simulink model "MotorControl"  (R2018b)
settings: Solver=FixedStepAuto  StartTime=0.0  StopTime=0.8  FixedStep=0.001  RelTol=1e-3  EnableMultiTasking=on
PostLoadFcn:
  | PMSM_Params
values from neighbouring files (symbols this model uses):
  Params =     [Parameters.mat]
libraries: TIMERS_Lib x3, ADC_Lib x2, USART_Lib x2, GPIO_Lib x1, STM32_Config_Lib x1
settings Model: DataTypeOverride=Double  MinMaxOverflowLogging=ForceOff  Creator=Alex  LastModifiedBy=fenard1
settings DataIOCC: LimitDataPoints=on  SaveFormat=Array
settings OptimizationCC: DefaultParameterBehavior=Inlined  DefaultUnderspecifiedDataType=single  PassReuseOutputArgsAs=Individual arguments  ExpressionDepthLimit=2147483647  LifeSpan=1
settings DebuggingCC: UnderspecifiedInitializationDetection=Classic  MergeDetectMultiDrivingBlocksExec=none  SolverPrmCheckMsg=warning  MultiTaskDSMMsg=none  UniqueDataStoreMsg=error  AllowSymbolicDim=off  StateNameClashWarn=warning  StrictBusMsg=ErrorOnBusTreatedAsVector  SFUnexpectedBacktrackingDiag=warning  SFNoUnconditionalDefaultTransitionDiag=warning  SFUndirectedBroadcastEventsDiag=error  SFExecutionAtInitializationDiag=none
settings HardwareCC: ProdBitPerPointer=32  ProdBitPerSizeT=32  ProdBitPerPtrDiffT=32  ProdLargestAtomicInteger=Integer  ProdWordSize=32  ProdHWDeviceType=STMicroelectronics->STM32 32-bit Cortex-M  TargetLargestAtomicInteger=Integer  TargetLargestAtomicFloat=Float  TargetIntDivRoundTo=Zero  TargetEndianess=LittleEndian  TargetHWDeviceType=STMicroelectronics->STM32F4xx 32-bit Cortex-M4
settings ModelReferenceCC: PropagateSignalLabelsOutOfModel=off
settings SFSimCC: SimUseLocalCustomCode=off  CompileTimeRecursionLimit=0  EnableRuntimeRecursion=off  MATLABDynamicMemAlloc=off
settings RTWCC: SystemTargetFile=stm32.tlc  TemplateMakefile=stm32.tmf  Description=stm32 (Embedded Target)  GenerateReport=on  RTWUseLocalCustomCode=off  IncludeHyperlinkInReport=on  GenerateCodeReplacementReport=on
settings CodeAppCC: IgnoreCustomStorageClasses=off  CustomSymbolStrType=$N$R$M  SimulinkBlockComments=off  InternalIdentifier=Classic
settings STFCustomTargetCC: TargetLangStandard=C99 (ISO)  CodeReplacementLibrary=ARM CMSIS SIN COS  ParMdlRefBuildCompliant=on  IncludeMdlTerminateFcn=off  CombineOutputUpdateFcns=on  ERTCustomFileBanners=on  SupportComplex=off  SupportContinuousTime=off  SupportNonInlinedSFcns=off  RemoveResetFunc=on  ParenthesesLevel=Maximum  CastingMode=Standards  MATLABClassNameForMDSCustomization=Simulink.SoftwareTarget.ERTCustomization  SystemTargetFile=stm32.tlc
settings ERTTargetCC: TargetLangStandard=C99 (ISO)  CodeReplacementLibrary=ARM CMSIS SIN COS  MultiwordLength=2048  CompOptLevelCompliant=off  ConcurrentExecutionCompliant=off  IncludeMdlTerminateFcn=off  SupportComplex=off  ParenthesesLevel=Maximum  CastingMode=Standards  ModelStepFunctionPrototypeControlCompliant=off  CPPClassGenCompliant=off  UseToolchainInfoCompliant=off  InlinedParameterPlacement=NonHierarchical  ERTSrcFileBannerTemplate=sourceFileTemplate.cgt  ERTHdrFileBannerTemplate=sourceFileTemplate.cgt  ERTDataSrcFileTemplate=sourceFileTemplate.cgt  ERTDataHdrFileTemplate=sourceFileTemplate.cgt  ERTCustomFileTemplate=customRoutineProcess.tlc  ConvertIfToSwitch=off  SuppressUnreachableDefaultCases=off  EnableSignedLeftShifts=off  EnableSignedRightShifts=off
settings ConfigComp: CovMetricSettings=dw  CovHtmlReporting=on  CovSaveCumulativeToWorkspaceVar=on  CovSaveSingleToWorkspaceVar=on  CovExternalEMLEnable=off  CovSFcnEnable=off
settings SimscapeCC: SimscapeNormalizeSystem=off

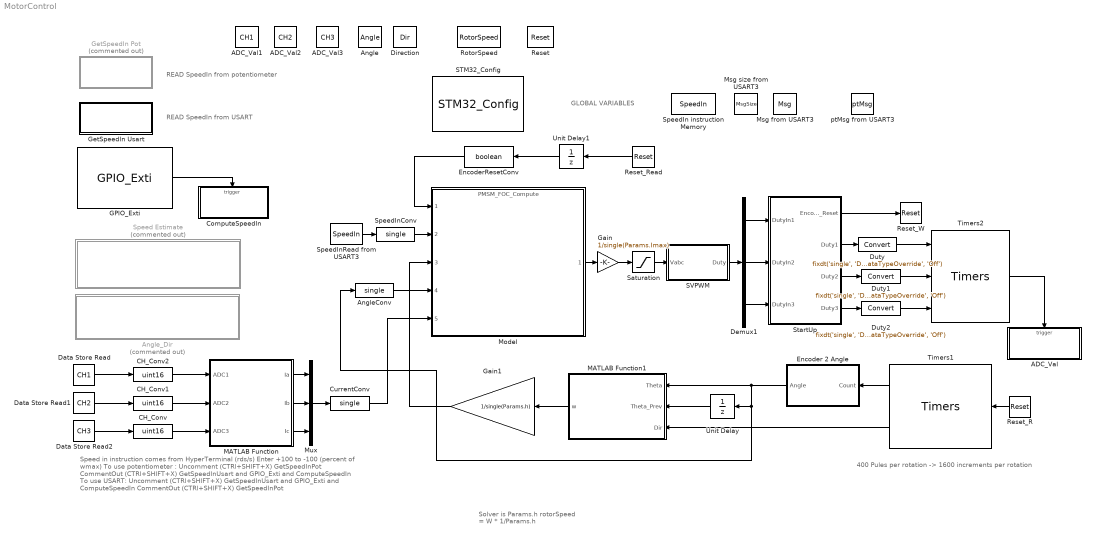
== system MotorControl ==
  note: Speed in instruction comes from HyperTerminal (rds/s)
      | Enter +100 to -100 (percent of wmax)
      | To use potentiometer :
      | Uncomment (CTRl+SHIFT+X) GetSpeedInPot
      | CommentOut (CTRl+SHIFT+X) GetSpeedInUsart and GPIO_Exti
      | and ComputeSpeedIn
      | To use USART:
      | Uncomment (CTRl+SHIFT+X) GetSpeedInUsart and GPIO_Exti
      | and ComputeSpeedIn
      | CommentOut (CTRl+SHIFT+X) GetSpeedInPot
  note: GLOBAL VARIABLES
  note: READ SpeedIn from potentiometer
  note: READ SpeedIn from USART
  note: 400 Pules per rotation -> 1600 increments per rotation
  note: Solver is Params.h
      | rotorSpeed = W * 1/Params.h
  ADC_Val : Subsystem  TreatAsAtomicUnit=on
  ADC_Val1 : DataStoreMemory  DataStoreName=CH1  ReadBeforeWriteMsg=warning  WriteAfterWriteMsg=warning  WriteAfterReadMsg=warning  ShowAdditionalParam=off  OutMin=0  OutMax=4095  OutDataTypeStr=fixdt('uint16', 'DataTypeOverride', 'Off')
  ADC_Val2 : DataStoreMemory  DataStoreName=CH2  ReadBeforeWriteMsg=warning  WriteAfterWriteMsg=warning  WriteAfterReadMsg=warning  ShowAdditionalParam=off  OutMin=0  OutMax=4095  OutDataTypeStr=fixdt('uint16', 'DataTypeOverride', 'Off')
  ADC_Val3 : DataStoreMemory  DataStoreName=CH3  ReadBeforeWriteMsg=warning  WriteAfterWriteMsg=warning  WriteAfterReadMsg=warning  ShowAdditionalParam=off  OutMin=0  OutMax=4095  OutDataTypeStr=fixdt('uint16', 'DataTypeOverride', 'Off')
  Angle : DataStoreMemory  DataStoreName=Angle  ReadBeforeWriteMsg=warning  WriteAfterWriteMsg=warning  WriteAfterReadMsg=warning  ShowAdditionalParam=off  OutDataTypeStr=fixdt('single', 'DataTypeOverride', 'Off')
  AngleConv : DataTypeConversion  OutDataTypeStr=single
  Angle_Dir : Subsystem  Commented=on  TreatAsAtomicUnit=on  SystemSampleTime=0.001
  CH_Conv : DataTypeConversion  OutDataTypeStr=uint16
  CH_Conv1 : DataTypeConversion  OutDataTypeStr=uint16
  CH_Conv2 : DataTypeConversion  OutDataTypeStr=uint16
  ComputeSpeedIn : Subsystem  TreatAsAtomicUnit=on
  CurrentConv : DataTypeConversion  OutDataTypeStr=single
  Data Store Read : DataStoreRead  DataStoreName=CH1
  Data Store Read1 : DataStoreRead  DataStoreName=CH2
  Data Store Read2 : DataStoreRead  DataStoreName=CH3
  Demux1 : Demux  Outputs=3
  Direction : DataStoreMemory  DataStoreName=Dir  ReadBeforeWriteMsg=warning  WriteAfterWriteMsg=warning  WriteAfterReadMsg=warning  ShowAdditionalParam=off  OutDataTypeStr=fixdt('uint8', 'DataTypeOverride', 'Off')
  Duty : DataTypeConversion  OutDataTypeStr=fixdt('single', 'DataTypeOverride', 'Off')
  Duty1 : DataTypeConversion  OutDataTypeStr=fixdt('single', 'DataTypeOverride', 'Off')
  Duty2 : DataTypeConversion  OutDataTypeStr=fixdt('single', 'DataTypeOverride', 'Off')
  Encoder 2 Angle : MATLAB Function  TreatAsAtomicUnit=on
      settings: MinAlgLoopOccurrences=on
  EncoderResetConv : DataTypeConversion  OutDataTypeStr=boolean
  GPIO_Exti : GPIO_Lib/GPIO_Exti  Port_name=GPIOB  Pin_0=off  Pin_1=off  Pin_2=off  Pin_3=off  Pin_4=off  Pin_5=off  Pin_6=off  Pin_7=off  Pin_8=off  Pin_9=off  Pin_10=off  Pin_11=off  Pin_12=off  Pin_13=off  Pin_14=off  Pin_15=on  PinList=GPIOB15GPIOC13
      settings: SourceProductName=Target Support Package - STM32 Adapter
  Gain : Gain  Gain=1/single(Params.Imax)
  Gain1 : Gain  Gain=1/single(Params.h)  OutDataTypeStr=double
  GetSpeedIn Pot : Subsystem  Commented=on  TreatAsAtomicUnit=on  SystemSampleTime=0.1
  GetSpeedIn Usart : Subsystem  TreatAsAtomicUnit=on  SystemSampleTime=0.1
  MATLAB Function : MATLAB Function  TreatAsAtomicUnit=on
  MATLAB Function1 : MATLAB Function  TreatAsAtomicUnit=on
  Model : ModelReference  ModelNameDialog=PMSM_FOC_Compute.slx  SimulationMode=Normal  ModelReferenceVersion=1.373
  Msg from USART3 : DataStoreMemory  DataStoreName=Msg  ReadBeforeWriteMsg=warning  WriteAfterWriteMsg=warning  WriteAfterReadMsg=warning  InitialValue=[0,0,0,0,0,0,0,0]  ShowAdditionalParam=off  OutDataTypeStr=fixdt('uint8', 'DataTypeOverride', 'Off')
  Msg size from USART3 : DataStoreMemory  DataStoreName=MsgSize  ReadBeforeWriteMsg=warning  WriteAfterWriteMsg=warning  WriteAfterReadMsg=warning  ShowAdditionalParam=off  OutDataTypeStr=fixdt('uint16', 'DataTypeOverride', 'Off')
  Mux : Mux  Inputs=3
  Reset : DataStoreMemory  DataStoreName=Reset  ReadBeforeWriteMsg=warning  WriteAfterWriteMsg=warning  WriteAfterReadMsg=warning  InitialValue=1  ShowAdditionalParam=off  OutDataTypeStr=fixdt('uint8', 'DataTypeOverride', 'Off')
  Reset_R : DataStoreRead  DataStoreName=Reset
  Reset_Read : DataStoreRead  DataStoreName=Reset
  Reset_W : DataStoreWrite  DataStoreName=Reset
  RotorSpeed : DataStoreMemory  DataStoreName=RotorSpeed  ReadBeforeWriteMsg=warning  WriteAfterWriteMsg=warning  WriteAfterReadMsg=warning  ShowAdditionalParam=off  OutDataTypeStr=fixdt('single', 'DataTypeOverride', 'Off')
  STM32_Config : STM32_Config_Lib/STM32_Config  Priority=0  Project_Path=.\  Config_File=STM32F302R_NUCLEO.ioc  MCU_Name=STM32F302R8Tx
      settings: SourceProductName=Target Support Package - STM32 Adapter
  SVPWM : MATLAB Function  TreatAsAtomicUnit=on
  Saturation : Saturate  UpperLimit=1  LowerLimit=-1
  Speed Estimate : Subsystem  Commented=on  TreatAsAtomicUnit=on  SystemSampleTime=1/500
  SpeedIn instruction Memory : DataStoreMemory  DataStoreName=SpeedIn  ReadBeforeWriteMsg=warning  WriteAfterWriteMsg=warning  WriteAfterReadMsg=warning  ShowAdditionalParam=off  OutMin=-100  OutMax=+100  OutDataTypeStr=fixdt('single', 'DataTypeOverride', 'Off')
  SpeedInConv : DataTypeConversion  OutDataTypeStr=single
  SpeedInRead from USART3 : DataStoreRead  DataStoreName=SpeedIn
  StartUp : Stateflow chart  TreatAsAtomicUnit=on
      settings: MinAlgLoopOccurrences=on
  Timers1 : TIMERS_Lib/Timers  currentTIM=TIM2  TIM_Name=TIM2  sysUsingTimer=off  TIM_APBClock=72000000  TIM_Set_Clk=off  TIM_Prescaler=0  TIM_Clock=72000000.00  Variable_frequency=off  TIM_Set_OutFreq=off  TIM_ARR=799  Output_frequency=90112.64  Repetition_counter=0  TIM_Mode=Up  TIM_DMA=none  TIM_IRQ=off  TIM_IRQ_ONLY=off  TIM_UP=off  TIM_TRG=off  TIM_COM=off  TIM_BRK=off  NbTIM=2  CH1_enable=on  CH1N_enable=off  CH1_type=Input_Encoder  CH1_DMA=off  CH1_int=off  CH1_edge=Rising  CH1_div=1  CH1_variable_duty=off  CH1_set_pulse=off  CH1_output_duty=0.00  CH1_pulse=0  CH2_enable=on  CH2N_enable=off  CH2_type=Input_Encoder  CH2_DMA=off  CH2_int=off  CH2_edge=Rising  CH2_div=1  CH2_variable_duty=off  CH2_set_pulse=off  CH2_output_duty=0.00  CH2_pulse=0  CH3_enable=off  CH3N_enable=off  CH3_type=Unknown  CH3_DMA=off  CH3_int=off  CH3_edge=Rising  CH3_div=1  CH3_variable_duty=off  CH3_set_pulse=off  CH3_output_duty=0.00  CH3_pulse=0  CH4_enable=off  CH4N_enable=off  CH4_type=Unknown  CH4_DMA=off  CH4_int=off  CH4_edge=Rising  CH4_div=1  CH4_variable_duty=off  CH4_set_pulse=off  CH4_output_duty=0.00  CH4_pulse=0
      settings: SourceProductName=Target Support Package - STM32 Adapter
  Timers2 : TIMERS_Lib/Timers  currentTIM=TIM1  TIM_Name=TIM1  sysUsingTimer=off  TIM_APBClock=72000000  TIM_Set_Clk=off  TIM_Prescaler=0  TIM_Clock=72000000.00  Variable_frequency=off  TIM_Set_OutFreq=on  TIM_ARR=7200  Output_frequency=10000.00  Repetition_counter=0  TIM_Mode=Center_Aligned_2  TIM_DMA=none  TIM_IRQ=off  TIM_IRQ_ONLY=off  TIM_UP=on  TIM_TRG=off  TIM_COM=off  TIM_BRK=off  NbTIM=2  CH1_enable=on  CH1N_enable=on  CH1_type=Output_PWM  CH1_DMA=off  CH1_int=off  CH1_edge=Rising  CH1_div=1  CH1_variable_duty=on  CH1_set_pulse=off  CH1_output_duty=30.00  CH1_pulse=2160  CH2_enable=on  CH2N_enable=on  CH2_type=Output_PWM  CH2_DMA=off  CH2_int=off  CH2_edge=Rising  CH2_div=1  CH2_variable_duty=on  CH2_set_pulse=off  CH2_output_duty=0.00  CH2_pulse=0  CH3_enable=on  CH3N_enable=on  CH3_type=Output_PWM  CH3_DMA=off  CH3_int=off  CH3_edge=Rising  CH3_div=1  CH3_variable_duty=on  CH3_set_pulse=off  CH3_output_duty=5.00  CH3_pulse=360  CH4_enable=off  CH4N_enable=off  CH4_type=Unknown  CH4_DMA=off  CH4_int=off  CH4_edge=Rising  CH4_div=1  CH4_variable_duty=off  CH4_set_pulse=off  CH4_output_duty=0.00  CH4_pulse=0
      settings: SourceProductName=Target Support Package - STM32 Adapter
  Unit Delay : UnitDelay  SampleTime=-1
  Unit Delay1 : UnitDelay  SampleTime=-1
  ptMsg from USART3 : DataStoreMemory  DataStoreName=ptMsg  ReadBeforeWriteMsg=warning  WriteAfterWriteMsg=warning  WriteAfterReadMsg=warning  ShowAdditionalParam=off  OutDataTypeStr=fixdt('uint32', 'DataTypeOverride', 'Off')
  wires:
  Demux1/1 -> StartUp/1(DutyIn1)
  Demux1/2 -> StartUp/2(DutyIn2)
  Demux1/3 -> StartUp/3(DutyIn3)
  StartUp/1(Encoder_Reset) -> Reset_W/1
  StartUp/2(Duty1) -> Duty/1
  Gain/1 -> Saturation/1
  Unit Delay1/1 -> EncoderResetConv/1
  EncoderResetConv/1 -> Model/1
  AngleConv/1 -> Model/4
  GPIO_Exti/1 -> ComputeSpeedIn/Trigger
  SpeedInRead from USART3/1 -> SpeedInConv/1
  SpeedInConv/1 -> Model/2
  StartUp/3(Duty2) -> Duty1/1
  StartUp/4(Duty3) -> Duty2/1
  Data Store Read/1 -> CH_Conv2/1
  Data Store Read1/1 -> CH_Conv1/1
  Reset_Read/1 -> Unit Delay1/1
  Timers1/1 -> Encoder 2 Angle/1(Count)
  Reset_R/1 -> Timers1/1
  Unit Delay/1 -> MATLAB Function1/2(Theta_Prev)
  MATLAB Function1/1(w) -> Gain1/1
  Timers1/2 -> MATLAB Function1/3(Dir)
  Encoder 2 Angle/1(Angle) -> AngleConv/1, Unit Delay/1, MATLAB Function1/1(Theta)
  Gain1/1 -> Model/3
  MATLAB Function/1(Ia) -> Mux/1
  MATLAB Function/2(Ib) -> Mux/2
  MATLAB Function/3(Ic) -> Mux/3
  Mux/1 -> CurrentConv/1
  CurrentConv/1 -> Model/5
  Model/1 -> Gain/1
  Saturation/1 -> SVPWM/1(Vabc)
  CH_Conv/1 -> MATLAB Function/3(ADC3)
  CH_Conv1/1 -> MATLAB Function/2(ADC2)
  CH_Conv2/1 -> MATLAB Function/1(ADC1)
  SVPWM/1(Duty) -> Demux1/1
  Duty/1 -> Timers2/1
  Duty2/1 -> Timers2/3
  Duty1/1 -> Timers2/2
  Data Store Read2/1 -> CH_Conv/1
  Timers2/1 -> ADC_Val/Trigger

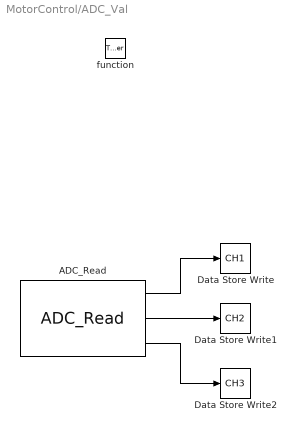
== system MotorControl/ADC_Val ==
  function : TriggerPort  TriggerType=function-call  VariantControl=Variant
  ADC_Read : ADC_Lib/ADC_Read  ADC_Name=ADC1  ADC_Ch0=off  ADC_Ch1=off  ADC_Ch2=off  ADC_Ch3=off  ADC_Ch4=off  ADC_Ch5=off  ADC_Ch6=off  ADC_Ch7=off  ADC_Ch8=on  ADC_Ch9=on  ADC_Ch10=on  ADC_Ch11=off  ADC_Ch12=off  ADC_Ch13=off  ADC_Ch14=off  ADC_Ch15=off  ADC_Ch16=off  ADC_Ch17=off  ADC_Ch18=off  RgRk1=on  RgRk2=on  RgRk3=on  RgRk4=off  RgRk1_Ch=Ch8_r1  RgRk2_Ch=Ch9_r2  RgRk3_Ch=Ch10_r3  RgRk4_Ch=off  RgRk5=off  RgRk6=off  RgRk7=off  RgRk8=off  RgRk5_Ch=off  RgRk6_Ch=off  RgRk7_Ch=off  RgRk8_Ch=off  RgRk9=off  RgRk10=off  RgRk11=off  RgRk12=off  RgRk9_Ch=off  RgRk10_Ch=off  RgRk11_Ch=off  RgRk12_Ch=off  RgRk13=off  RgRk14=off  RgRk15=off  RgRk16=off  RgRk13_Ch=off  RgRk14_Ch=off  RgRk15_Ch=off  RgRk16_Ch=off  InjRk1=off  InjRk2=off  InjRk3=off  InjRk4=off  InjRk1_Ch=off  InjRk2_Ch=off  InjRk3_Ch=off  InjRk4_Ch=off  ADC_Trig=T1_TRGO  ADC_TrigEdge=RISING  DmaReq=on  DMA_Buffer=128  ItReq=off  AWD_Mode=NOT_USED  AWD_Ch=0  AWD_HThres=0  AWD_LThres=0  AWD_En_Int=off  AWD2_HThres=0  AWD2_LThres=0  AWD2_En_Int=off  AWD3_HThres=0  AWD3_LThres=0  AWD3_En_Int=off  EOC_SEQ=off  EOC_IT=off  JEOC_IT=off  AWD_IT=off  OVR_IT=off  CpltTrans=off  HalfTrans=off  ADC_RegNb=3  ADC_RegCh0=off  ADC_RegCh1=off  ADC_RegCh2=off  ADC_RegCh3=off  ADC_RegCh4=off  ADC_RegCh5=off  ADC_RegCh6=off  ADC_RegCh7=off  ADC_RegCh8=on  ADC_RegCh9=on  ADC_RegCh10=on  ADC_RegCh11=off  ADC_RegCh12=off  ADC_RegCh13=off  ADC_RegCh14=off  ADC_RegCh15=off  ADC_RegCh16=off  ADC_RegCh17=off  ADC_RegCh18=off  ADC_InjNb=0  ADC_InjCh0=off  ADC_InjCh1=off  ADC_InjCh2=off  ADC_InjCh3=off  ADC_InjCh4=off  ADC_InjCh5=off  ADC_InjCh6=off  ADC_InjCh7=off  ADC_InjCh8=off  ADC_InjCh9=off  ADC_InjCh10=off  ADC_InjCh11=off  ADC_InjCh12=off  ADC_InjCh13=off  ADC_InjCh14=off  ADC_InjCh15=off  ADC_InjCh16=off  ADC_InjCh17=off  ADC_InjCh18=off  NbADC=1  CurrentADC=ADC1
      settings: SourceProductName=Target Support Package - STM32 Adapter
  Data Store Write : DataStoreWrite  DataStoreName=CH1
  Data Store Write1 : DataStoreWrite  DataStoreName=CH2
  Data Store Write2 : DataStoreWrite  DataStoreName=CH3
  wires:
  ADC_Read/3 -> Data Store Write2/1
  ADC_Read/1 -> Data Store Write/1
  ADC_Read/2 -> Data Store Write1/1

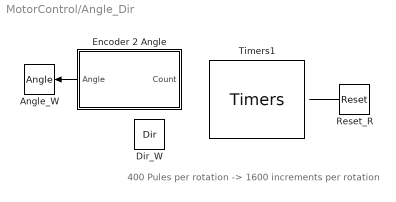
== system MotorControl/Angle_Dir ==
  note: 400 Pules per rotation -> 1600 increments per rotation
  Angle_W : DataStoreWrite  DataStoreName=Angle
  Dir_W : DataStoreWrite  DataStoreName=Dir
  Encoder 2 Angle : MATLAB Function  TreatAsAtomicUnit=on
      settings: MinAlgLoopOccurrences=on
  Reset_R : DataStoreRead  DataStoreName=Reset
  Timers1 : TIMERS_Lib/Timers  currentTIM=none  TIM_Name=TIM1  sysUsingTimer=on  TIM_APBClock=96000000  TIM_Set_Clk=off  TIM_Prescaler=2  TIM_Clock=24000000.00  Variable_frequency=off  TIM_Set_OutFreq=off  TIM_ARR=799  Output_frequency=30037.55  Repetition_counter=0  TIM_Mode=Up  TIM_DMA=none  TIM_IRQ=off  TIM_IRQ_ONLY=on  TIM_UP=off  TIM_TRG=off  TIM_COM=off  TIM_BRK=off  NbTIM=2  CH1_enable=off  CH1N_enable=off  CH1_type=Output_PWM  CH1_DMA=off  CH1_int=off  CH1_edge=Rising  CH1_div=1  CH1_variable_duty=off  CH1_set_pulse=off  CH1_output_duty=0.00  CH1_pulse=0  CH2_enable=off  CH2N_enable=off  CH2_type=Output_PWM  CH2_DMA=off  CH2_int=off  CH2_edge=Rising  CH2_div=1  CH2_variable_duty=off  CH2_set_pulse=off  CH2_output_duty=0.00  CH2_pulse=0  CH3_enable=off  CH3N_enable=off  CH3_type=Output_PWM  CH3_DMA=off  CH3_int=off  CH3_edge=Rising  CH3_div=1  CH3_variable_duty=off  CH3_set_pulse=off  CH3_output_duty=0.00  CH3_pulse=0  CH4_enable=off  CH4N_enable=off  CH4_type=Unknown  CH4_DMA=off  CH4_int=off  CH4_edge=Rising  CH4_div=1  CH4_variable_duty=off  CH4_set_pulse=off  CH4_output_duty=0.00  CH4_pulse=0
      settings: SourceProductName=Target Support Package - STM32 Adapter
  wires:
  Encoder 2 Angle/1(Angle) -> Angle_W/1
  ? -> Dir_W/1
  ? -> Encoder 2 Angle/1(Count)
  Reset_R/1 -> ?

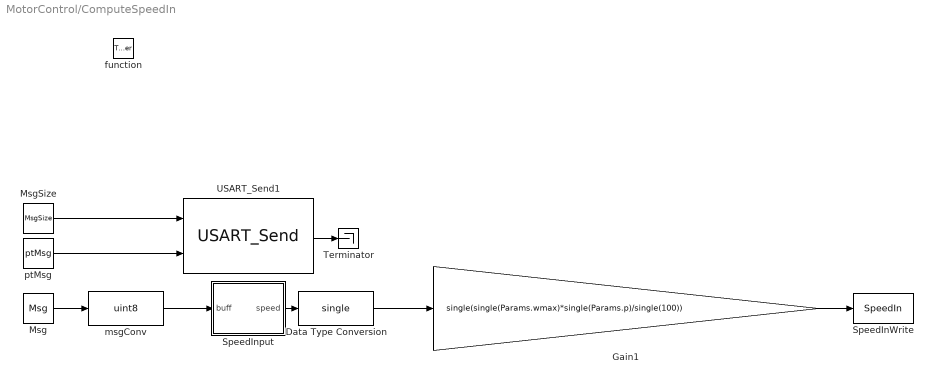
== system MotorControl/ComputeSpeedIn ==
  function : TriggerPort  TriggerType=function-call  VariantControl=Variant
  Data Type Conversion : DataTypeConversion  OutDataTypeStr=single
  Gain1 : Gain  Gain=single(single(Params.wmax)*single(Params.p)/single(100))  ParamDataTypeStr=double  OutDataTypeStr=fixdt('single', 'DataTypeOverride', 'Off')
  Msg : DataStoreRead  DataStoreName=Msg
  MsgSize : DataStoreRead  DataStoreName=MsgSize
  SpeedInWrite : DataStoreWrite  DataStoreName=SpeedIn
  SpeedInput : MATLAB Function  TreatAsAtomicUnit=on
  Terminator : Terminator
  USART_Send1 : USART_Lib/USART_Send  USART_name=USART2  Buff_size=16  nbUsart=1  usartMode=Asynchronous  usartDma_Rx=off  usartDma_Tx=off  usartIt=on
      settings: SourceProductName=Target Support Package - STM32 Adapter
  msgConv : DataTypeConversion  OutDataTypeStr=uint8
  ptMsg : DataStoreRead  DataStoreName=ptMsg
  wires:
  Msg/1 -> msgConv/1
  MsgSize/1 -> USART_Send1/1
  SpeedInput/1(speed) -> Data Type Conversion/1
  Data Type Conversion/1 -> Gain1/1
  Gain1/1 -> SpeedInWrite/1
  ptMsg/1 -> USART_Send1/2
  msgConv/1 -> SpeedInput/1(buff)
  USART_Send1/1 -> Terminator/1

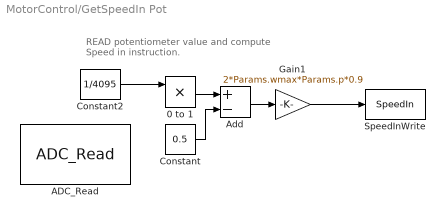
== system MotorControl/GetSpeedIn Pot ==
  note: READ potentiometer value and
      | compute Speed in instruction.
  0 to 1 : Product  OutMin=0  OutMax=1  OutDataTypeStr=double  RndMeth=Zero
  ADC_Read : ADC_Lib/ADC_Read  ADC_Name=ADC1  ADC_Ch0=off  ADC_Ch1=off  ADC_Ch2=off  ADC_Ch3=off  ADC_Ch4=off  ADC_Ch5=off  ADC_Ch6=off  ADC_Ch7=off  ADC_Ch8=off  ADC_Ch9=off  ADC_Ch10=off  ADC_Ch11=off  ADC_Ch12=off  ADC_Ch13=off  ADC_Ch14=off  ADC_Ch15=off  ADC_Ch16=off  ADC_Ch17=off  ADC_Ch18=off  RgRk1=off  RgRk2=off  RgRk3=off  RgRk4=off  RgRk1_Ch=Ch8_r1  RgRk2_Ch=Ch9_r2  RgRk3_Ch=Ch10_r3  RgRk4_Ch=off  RgRk5=off  RgRk6=off  RgRk7=off  RgRk8=off  RgRk5_Ch=off  RgRk6_Ch=off  RgRk7_Ch=off  RgRk8_Ch=off  RgRk9=off  RgRk10=off  RgRk11=off  RgRk12=off  RgRk9_Ch=off  RgRk10_Ch=off  RgRk11_Ch=off  RgRk12_Ch=off  RgRk13=off  RgRk14=off  RgRk15=off  RgRk16=off  RgRk13_Ch=off  RgRk14_Ch=off  RgRk15_Ch=off  RgRk16_Ch=off  InjRk1=off  InjRk2=off  InjRk3=off  InjRk4=off  InjRk1_Ch=off  InjRk2_Ch=off  InjRk3_Ch=off  InjRk4_Ch=off  ADC_Trig=T1_TRGO  ADC_TrigEdge=RISING  DmaReq=on  DMA_Buffer=128  ItReq=off  AWD_Mode=NOT_USED  AWD_Ch=0  AWD_HThres=0  AWD_LThres=0  AWD_En_Int=off  AWD2_HThres=0  AWD2_LThres=0  AWD2_En_Int=off  AWD3_HThres=0  AWD3_LThres=0  AWD3_En_Int=off  EOC_SEQ=off  EOC_IT=off  JEOC_IT=off  AWD_IT=off  OVR_IT=off  CpltTrans=off  HalfTrans=off  ADC_RegNb=3  ADC_RegCh0=off  ADC_RegCh1=off  ADC_RegCh2=off  ADC_RegCh3=off  ADC_RegCh4=off  ADC_RegCh5=off  ADC_RegCh6=off  ADC_RegCh7=off  ADC_RegCh8=on  ADC_RegCh9=on  ADC_RegCh10=on  ADC_RegCh11=off  ADC_RegCh12=off  ADC_RegCh13=off  ADC_RegCh14=off  ADC_RegCh15=off  ADC_RegCh16=off  ADC_RegCh17=off  ADC_RegCh18=off  ADC_InjNb=0  ADC_InjCh0=off  ADC_InjCh1=off  ADC_InjCh2=off  ADC_InjCh3=off  ADC_InjCh4=off  ADC_InjCh5=off  ADC_InjCh6=off  ADC_InjCh7=off  ADC_InjCh8=off  ADC_InjCh9=off  ADC_InjCh10=off  ADC_InjCh11=off  ADC_InjCh12=off  ADC_InjCh13=off  ADC_InjCh14=off  ADC_InjCh15=off  ADC_InjCh16=off  ADC_InjCh17=off  ADC_InjCh18=off  ADC_RegRank0=0  ADC_RegRank1=0  ADC_RegRank2=0  ADC_RegRank3=0  ADC_RegRank4=0  ADC_RegRank5=0  ADC_RegRank6=0  ADC_RegRank7=0  ADC_RegRank8=1  ADC_RegRank9=2  ADC_RegRank10=3  ADC_RegRank11=0  ADC_RegRank12=0  ADC_RegRank13=0  ADC_RegRank14=0  ADC_RegRank15=0  ADC_RegRank16=0  ADC_RegRank17=0  ADC_RegRank18=0  ADC_InjRank0=0  ADC_InjRank1=0  ADC_InjRank2=0  ADC_InjRank3=0  ADC_InjRank4=0  ADC_InjRank5=0  ADC_InjRank6=0  ADC_InjRank7=0  ADC_InjRank8=0  ADC_InjRank9=0  ADC_InjRank10=0  ADC_InjRank11=0  ADC_InjRank12=0  ADC_InjRank13=0  ADC_InjRank14=0  ADC_InjRank15=0  ADC_InjRank16=0  ADC_InjRank17=0  ADC_InjRank18=0  NbADC=1  CurrentADC=ADC1
      settings: SourceProductName=Target Support Package - STM32 Adapter
  Add : Sum  Inputs=+-  AccumDataTypeStr=double  OutMin=-0.5  OutMax=0.5
  Constant : Constant  Value=0.5
  Constant2 : Constant  Value=1/4095
  Gain1 : Gain  Gain=2*Params.wmax*Params.p*0.9  ParamDataTypeStr=double  OutDataTypeStr=double
  SpeedInWrite : DataStoreWrite  DataStoreName=SpeedIn
  wires:
  0 to 1/1 -> Add/1
  ? -> 0 to 1/2
  Constant2/1 -> 0 to 1/1
  Constant/1 -> Add/2
  Add/1 -> Gain1/1
  Gain1/1 -> SpeedInWrite/1

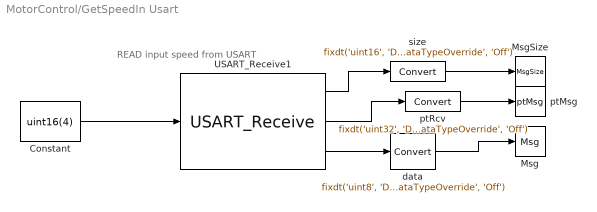
== system MotorControl/GetSpeedIn Usart ==
  note: READ input speed from USART
  Constant : Constant  Value=uint16(4)  OutDataTypeStr=fixdt('uint16', 'DataTypeOverride', 'Off')
  Msg : DataStoreWrite  DataStoreName=Msg
  MsgSize : DataStoreWrite  DataStoreName=MsgSize
  USART_Receive1 : USART_Lib/USART_Receive  USART_name=USART2  Buff_size=8  nbUsart=1  Soft_it=on  Soft_num=15  usartMode=Asynchronous  usartDma_Rx=off  usartDma_Tx=off  usartIt=on
      settings: SourceProductName=Target Support Package - STM32 Adapter
  data : DataTypeConversion  OutDataTypeStr=fixdt('uint8', 'DataTypeOverride', 'Off')
  ptMsg : DataStoreWrite  DataStoreName=ptMsg
  ptRcv : DataTypeConversion  OutDataTypeStr=fixdt('uint32', 'DataTypeOverride', 'Off')
  size : DataTypeConversion  OutDataTypeStr=fixdt('uint16', 'DataTypeOverride', 'Off')
  wires:
  Constant/1 -> USART_Receive1/1
  USART_Receive1/2 -> ptRcv/1
  USART_Receive1/3 -> data/1
  USART_Receive1/1 -> size/1
  size/1 -> MsgSize/1
  ptRcv/1 -> ptMsg/1
  data/1 -> Msg/1

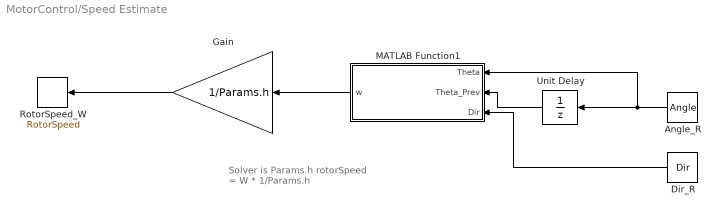
== system MotorControl/Speed Estimate ==
  note: Solver is Params.h
      | rotorSpeed = W * 1/Params.h
  Angle_R : DataStoreRead  DataStoreName=Angle
  Dir_R : DataStoreRead  DataStoreName=Dir
  Gain : Gain  Gain=1/Params.h  OutDataTypeStr=double
  MATLAB Function1 : MATLAB Function  TreatAsAtomicUnit=on
  RotorSpeed_W : DataStoreWrite  DataStoreName=RotorSpeed
  Unit Delay : UnitDelay  SampleTime=-1
  wires:
  Unit Delay/1 -> MATLAB Function1/2(Theta_Prev)
  MATLAB Function1/1(w) -> Gain/1
  Angle_R/1 -> MATLAB Function1/1(Theta), Unit Delay/1
  Dir_R/1 -> MATLAB Function1/3(Dir)
  Gain/1 -> RotorSpeed_W/1

== stateflow chart MotorControl/StartUp ==
  state Startup
    entry: Encoder_Reset = uint8(1);
    Duty1 = single(30);
    Duty2 =single(-1);
    Duty3 = single(5);
  state Running
    entry: Encoder_Reset = uint8(0);
    Duty1 = single(DutyIn1);
    Duty2 = single(DutyIn2);
    Duty3 = single(DutyIn3);
  (default) -> Startup
  Startup -> Running : [after(0.2,sec)]
  Running -> Running : [1]
  data: Encoder_Reset output fixdt('uint8', 'DataTypeOverride', 'Off') size=1; DutyIn1 input single size=1; DutyIn2 input single size=1; DutyIn3 input single size=1; Duty1 output fixdt('single', 'DataTypeOverride', 'Off') size=1; Duty2 output fixdt('single', 'DataTypeOverride', 'Off') size=1; Duty3 output fixdt('single', 'DataTypeOverride', 'Off') size=1

== matlab function MotorControl/Angle_Dir/Encoder 2 Angle ==
  data: Count input; Angle output; Params parameter
function Angle = Count2Angle(Count,Params)

Temp = cast(Count,'double');
Angle = (Temp*Params.Encoder_Gain+Params.Theta_Zero);
Angle = mod(Angle,2*pi);
end

== matlab function MotorControl/MATLAB Function ==
  data: ADC1 input; ADC2 input; Ia output; ADC3 input; Ib output; Ic output
function [Ia,Ib,Ic] = Convert(ADC1,ADC2,ADC3)
% convert ADC output to amps (0.22 ohm resistors and gain of G=6.4)
% Vshunt = I*0.22*G 
% ADC out = Vshunt/3.3 * 4096
% I*0.22*G*4096/3.3
% I = ADC_out*3.3/0.22*G*4096
Offset = single(1.94);
G = single(6.4);
R = single(0.22);
Va = ((cast(ADC1,'single')*single(3.3)/single(4096))-Offset)/G;
Vb = ((cast(ADC2,'single')*single(3.3)/single(4096))-Offset)/G;
Vc = ((cast(ADC3,'single')*single(3.3)/single(4096))-Offset)/G;

Ia = -Va/R;
Ib = -Vb/R;
Ic = -Vc/R;

== matlab function MotorControl/ComputeSpeedIn/SpeedInput ==
  data: buff input; speed output
function speed = SpeedInput(buff)
if coder.target('Sfun')
    % Executing in MATLAB, Buff is null
    speed = int32(0);
else
    coder.cinclude('stdio.h');
    
    speed = int32(0);
    buff1 = char(buff);
    %speed = coder.ceval('atoi',coder.ref(buff));
    %coder.ceval('getBuffPtr',coder.ref(buff));
    coder.ceval('sscanf',coder.rref(buff1),'%d',coder.wref(speed));
end
end

== matlab function MotorControl/Speed Estimate/MATLAB Function1 ==
  data: Theta input; w output; Theta_Prev input; Dir input
function w = fcn(Theta,Theta_Prev,Dir)

% if Dir = 1 -> downcounting, Dir = 0 -> upcounting
if (Theta < Theta_Prev)&& (Dir == 0)
    % Positive Roll Over
    w = Theta+2*pi-Theta_Prev;
elseif (Theta > Theta_Prev)&& (Dir == 1)
    % Underflow
    w = Theta-2*pi-Theta_Prev;
else
    w = Theta-Theta_Prev;
end

== matlab function MotorControl/Encoder 2 Angle ==
  data: Count input; Angle output; Params parameter
function Angle = Count2Angle(Count,Params)

Temp = cast(Count,'single');
%Angle = (Temp*single(Params.Encoder_Gain)+single(Params.Theta_Zero));
Angle = (Temp*single(2*single(pi)/800)+single(Params.Theta_Zero));
Angle = mod(Angle,2*single(pi));
end

== matlab function MotorControl/SVPWM ==
  data: Vabc input; Duty output
function Duty = SVPWM(Vabc)

%A = Vabc;
%Duty = (A-(min(A)+max(A))*0.5)*2/sqrt(3);
%Duty = A*2/sqrt(3);
Duty = single(Vabc);
Duty = ((Duty+1)/2)*single(100); %Add 1 to go from -1;1 to 0;2 so /2 and must give percentage
if ( Duty(1) < 0)
    Duty(1) = single(0);
end
if ( Duty(2) < 0)
    Duty(2) = single(0);
end
if (Duty(3) < 0)
    Duty(3) =single(0);
end
if (Duty(1) > 100)
    Duty(1) = single(100);
end
if (Duty(2) > 100)
    Duty(2) = single(100);
end
if (Duty(3) > 100)
    Duty(3) = single(100);
end
;

== matlab function MotorControl/MATLAB Function1 ==
  data: Theta input; w output; Theta_Prev input; Dir input
function w = fcn(Theta,Theta_Prev,Dir)

% if Dir = 1 -> downcounting, Dir = 0 -> upcounting
if (Theta < Theta_Prev)&& (Dir == 0)
    % Positive Roll Over
    w = single(Theta)+2*single(pi)-single(Theta_Prev);
elseif (Theta > Theta_Prev)&& (Dir == 1)
    % Underflow
    w = single(Theta)-2*single(pi)-single(Theta_Prev);
else
    w = single(Theta)-single(Theta_Prev);
end
